simulink model "NewtonsLawOfCooling_SIM"  (R2012b)
settings: Solver=ode3  StartTime=0.0  StopTime=10.0  FixedStep=0.1  RelTol=1e-3
settings Model: Creator=aluno  LastModifiedBy=aluno
settings DataIOCC: Refine=10
settings DebuggingCC: SolverPrmCheckMsg=none

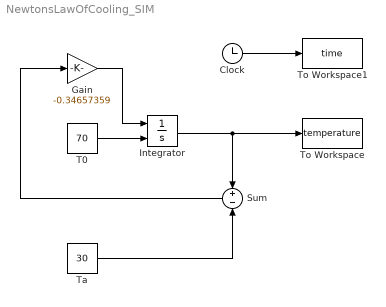
== system NewtonsLawOfCooling_SIM ==
  Clock : Clock
  Gain : Gain  Gain=-0.34657359
  Integrator : Integrator  InitialConditionSource=external
  Sum : Sum  Inputs=+-
  T0 : Constant  Value=70
  "Ta " : Constant  Value=30
  To Workspace : ToWorkspace  VariableName=temperature  SampleTime=-1
  To Workspace1 : ToWorkspace  VariableName=time  SampleTime=-1
  wires:
  Integrator/1 -> To Workspace/1, Sum/1
  "Ta "/1 -> Sum/2
  T0/1 -> Integrator/2
  Sum/1 -> Gain/1
  Gain/1 -> Integrator/1
  Clock/1 -> To Workspace1/1
